simulink model "pv_tilt_sunspot_wiper"  (R2020a)
settings: Solver=VariableStepAuto  StartTime=0.0  StopTime=0.01  FixedStep=1e-8  RelTol=1e-3
libraries: powerlib x4, sm_lib x3, re_lib x1
settings Model: Creator=Mahsa  LastModifiedBy=Mahsa
settings DebuggingCC: SolverPrmCheckMsg=warning  StateNameClashWarn=warning

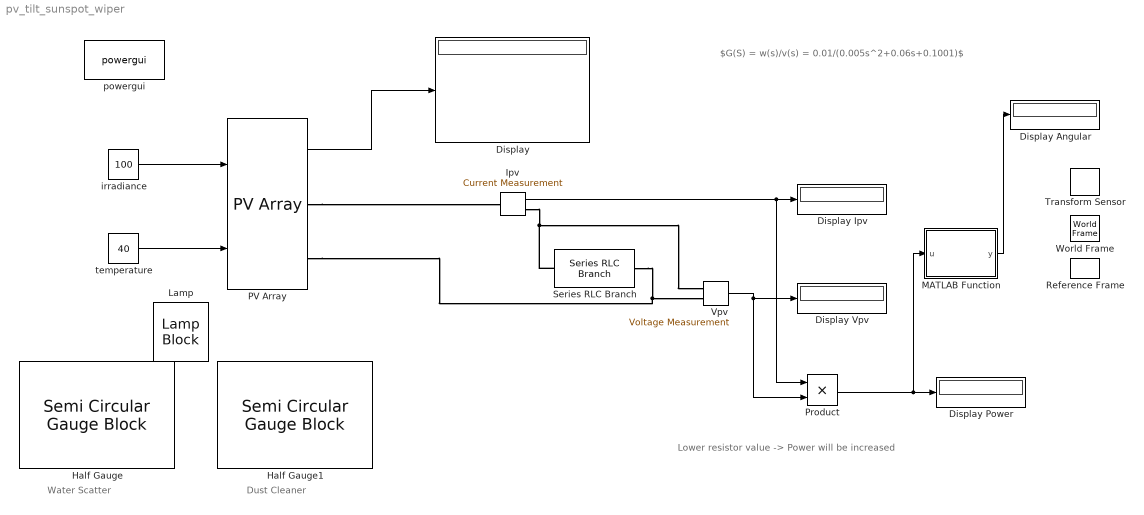
== system pv_tilt_sunspot_wiper ==
  note: Water Scatter
  note: $G(S) = w(s)/v(s) = 0.01/(0.005s^2+0.06s+0.1001)$
  note: Lower resistor value -> Power will be increased
  note: Dust Cleaner
  Display : Display
  Display Ipv : Display
  Display Power : Display
  Display Vpv : Display
  Display َAngular : Display
  Half Gauge : SemiCircularGaugeBlock
  Half Gauge1 : SemiCircularGaugeBlock
  Ipv : powerlib/Measurements/Current Measurement  PhasorSimulation=off  OutputType=Complex  PSBequivalent=0
  Lamp : LampBlock
  MATLAB Function : MATLAB Function  TreatAsAtomicUnit=on
  PV Array : re_lib/Solar/PV Array  Npar=40  Nser=10  PlotType=array @ 1000 W/m2 & specified temperatures  S_vec="[ 1000  500  100 ]"  Temp_C_vec="[ 45 25  ]"  ModuleName=1Soltech 1STH-215-P  PlotWhenSelected=off  Pm=213.15  Ncell=60  Voc=36.3  Isc=7.84  Vm=29  Im=7.35  beta_Voc_pc=-0.36099  alpha_Isc_pc=0.102  beta_Voc=-0.13104  alpha_Isc=0.007997  IL=7.8649  I0=2.9259e-10  nI=0.98117  Rsh=313.3991  Rs=0.39383  RobustModel=off  RobustCellTemperature=25  BAL=on  Tc=1e-6  Tfilter=5e-5
  Product : Product
  Reference Frame : sm_lib/Frames and Transforms/Reference Frame
  Series RLC Branch : powerlib/Elements/Series RLC Branch  LConnTagsString=__new0  RConnTagsString=__new0  BranchType=R  Resistance=4  Inductance=1e-3  SetiL0=off  InitialCurrent=0  Capacitance=1e-6  Setx0=off  InitialVoltage=0  Measurements=None
  Transform Sensor : sm_lib/Frames and Transforms/Transform Sensor  MeasurementFrame=World  SenseAngle=on  SenseAxis=off  SenseAngle1=off  SenseAngle2=off  SenseAngle3=off  SenseQ=off  SenseR=off  SenseOmegaX=off  SenseOmegaY=off  SenseOmegaZ=off  SenseOmega1=off  SenseOmega2=off  SenseOmega3=off  SenseQDot=off  SenseRDot=off  SenseAlphaX=off  SenseAlphaY=off  SenseAlphaZ=off  SenseAlpha1=off  SenseAlpha2=off  SenseAlpha3=off  SenseQDDot=off  SenseRDDot=off  SenseX=off  SenseY=off  SenseZ=off  SenseRad=off  SenseAzim=off  SenseDist=off  SenseInc=off  SenseXDot=off  SenseYDot=off  SenseZDot=off  SenseRadDot=off  SenseAzimDot=off  SenseDistDot=off  SenseIncDot=off  SenseXDDot=off  SenseYDDot=off  SenseZDDot=off  SenseRadDDot=off  SenseAzimDDot=off  SenseDistDDot=off  SenseIncDDot=off
  Vpv : powerlib/Measurements/Voltage Measurement  PhasorSimulation=off  OutputType=Complex  PSBequivalent=0
  World Frame : sm_lib/Frames and Transforms/World Frame
  irradiance : Constant  Value=100
  powergui : powerlib/powergui  Priority=1  SimulationMode=Discrete  SampleTime=1e-8  frequency=60  Iterations=50  frequencyindice=0  Pbase=100e6  ErrMax=1e-4  UnitsV=kV  UnitsW=MW  buscounter=0  FunctionMessages=off  echomessages=off  EnableUseOfTLC=off  CurrentSourceSwitches=off  DisableSnubberDevices=off  DisableRonSwitches=off  DisableVfSwitches=off  DisplayEquations=off  AutomaticDiscreteSolvers=off  SolverType=Tustin/Backward Euler (TBE)  Interpol=off  ExternalGateDelay=off  methode=off  Ts=100  x0status=blocks  SPID=on  SwTol=0  HookPort=off  NonlinearTolerance=1e-4  nMaxIteration=100  ContinueOnMaxIteration=off  RestoreLinks=warning  ResistiveCurrentMeasurement=off  Frange=[0:2:500]  Ylog=off  Xlog=on  ShowGrid=off  save=off  variable=ZData  structure=0  ZoomFFT=off  StartTime=0.0  cycles=1  DisplayStyle=1  fundamental=60  FreqAxis=off  MaxFrequency=1000  frequencyindicesteady=1  RmsSteady=1  display=off
  temperature : Constant  Value=40
  wires:
  Vpv/1 -> Product/2, Display Vpv/1
  irradiance/1 -> PV Array/1
  PV Array/1 -> Display/1
  Ipv/1 -> Product/1, Display Ipv/1
  temperature/1 -> PV Array/2
  Product/1 -> MATLAB Function/1(u), Display Power/1
  MATLAB Function/1(y) -> Display َAngular/1
  connections:
  PV Array/RConn2 -- Series RLC Branch/RConn1 -- Vpv/LConn2
  PV Array/RConn1 -- Ipv/LConn1
  Ipv/RConn1 -- Series RLC Branch/LConn1 -- Vpv/LConn1

== matlab function pv_tilt_sunspot_wiper/MATLAB Function ==
  data: u input; y output
function y = fcn(u)
u = 0.01/(0.005*u^2+0.06*u+0.1001);
y = u;
